simulink model "Ziegler4_27"  (Simulink 5.0)
settings: Solver=ode45  StartTime=0.0  StopTime=15  FixedStep=0.25  RelTol=1e-3
values from neighbouring files (symbols this model uses):
  kd = kp*pi/(4*wr)    [ZieglerDm4_29.m]    (also in Zieglerm4_27.m; example4_15.m = 0.01; example4_16.m = 0.006)
  ki = kp*wr/pi    [ZieglerDm4_29.m]    (also in Zieglerm4_27.m; example4_15.m = 1; example4_16.m = 0.01)
  kp = 0.6*kr    [ZieglerDm4_29.m]    (also in Zieglerm4_27.m; example4_15.m = 1.5; example4_16.m = 1.9)
libraries: simulink_extras x3
settings Model: LastModifiedBy=ThinkPad  ExtModeTrigMode=oneshot  ExtModeArmWhenConnect=off  LimitDataPoints=off  BooleanDataType=off

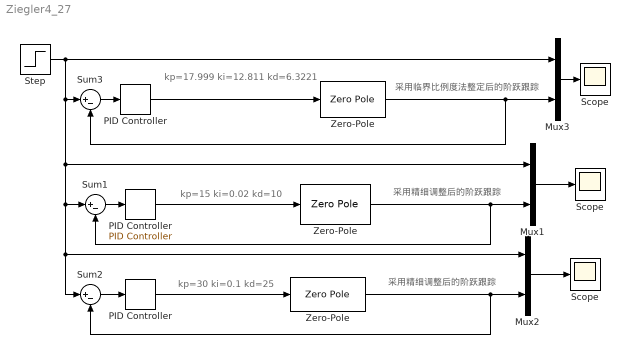
== system Ziegler4_27 ==
  note: 采用临界比例度法整定后的阶跃跟踪
  note: 采用精细调整后的阶跃跟踪
  note: kp=17.999 ki=12.811 kd=6.3221
  note: kp=15 ki=0.02 kd=10
  note: 采用精细调整后的阶跃跟踪
  note: kp=30 ki=0.1 kd=25
  " PID Controller " : simulink_extras/Additional Linear/PID Controller  P=15  I=0.02  D=10
  " Scope " : Scope
      settings: YMin=-3.5  YMax=1  MaxDataPoints=500000
  " Zero-Pole " : ZeroPole  Zeros=[]  Poles=[0 -1 -5]
  Mux1 : Mux  Inputs=2
  Mux2 : Mux  Inputs=2
  Mux3 : Mux  Inputs=2
  PID Controller : simulink_extras/Additional Linear/PID Controller  P=kp  I=ki  D=kd
  "PID Controller " : simulink_extras/Additional Linear/PID Controller  P=30  I=0.1  D=25
  Scope : Scope
      settings: YMin=-3.5  YMax=1  SaveName=Ziegler  DataFormat=Array  MaxDataPoints=500000
  "Scope " : Scope
      settings: YMin=-3.5  YMax=1  SaveName=ZieglerPID  DataFormat=Array  MaxDataPoints=500000
  Step : Step  Time=0  SampleTime=0
  Sum1 : Sum  Inputs=|+-  SaturateOnIntegerOverflow=on
  Sum2 : Sum  Inputs=|+-  SaturateOnIntegerOverflow=on
  Sum3 : Sum  Inputs=|+-  SaturateOnIntegerOverflow=on
  Zero-Pole : ZeroPole  Zeros=[]  Poles=[0 -1 -5]
  "Zero-Pole " : ZeroPole  Zeros=[]  Poles=[0 -1 -5]
  wires:
  Step/1 -> Mux3/1, Sum1/1, Mux2/1, Sum2/1, Mux1/1, Sum3/1
  Mux3/1 -> Scope/1
  "Zero-Pole "/1 -> Mux3/2, Sum3/2
  Sum3/1 -> PID Controller/1
  PID Controller/1 -> "Zero-Pole "/1
  Mux1/1 -> "Scope "/1
  Zero-Pole/1 -> Mux1/2, Sum1/2
  Sum1/1 -> " PID Controller "/1
  " PID Controller "/1 -> Zero-Pole/1
  " Zero-Pole "/1 -> Mux2/2, Sum2/2
  "PID Controller "/1 -> " Zero-Pole "/1
  Mux2/1 -> " Scope "/1
  Sum2/1 -> "PID Controller "/1
